simulink model "sensorMCU"  (Simulink 6.6)
settings: Solver=FixedStepDiscrete  StartTime=0.0  StopTime=10.0  FixedStep=0.01  RelTol=1e-3
InitFcn:
  | mcuInit
values from neighbouring files (symbols this model uses):
  gxGainrad = gxGain*pi/180    [mcuInit.m]
  gyGainrad = gyGain*pi/180    [mcuInit.m]
  gzGainrad = gzGain*pi/180    [mcuInit.m]
  T = 0.01    [initGPS.m]    (also in mcuInit.m)
undefined symbols (not defined in the file or in its folder): AccelParam, floatToBytes, gaind, gpsInit, gpsParse, gpsRead, gpsSeparate, gyTGain, hil_getEuler, hil_getGPSRead, hil_getRates, hil_getRawRead, hil_getVned, hil_getXYZ, hilRead, logData, loggerInit, MagParam, mzTGain, polesd, protParseDecode, protParserInit, shortToBytes, spiMasterInit, spiSend, stTGain, tmeanMz, tmeanSt, tmeanVl, u1, uartInit, uShortToBytes, vlTGain, y1, zerosd
libraries: dsPICdrivers x72, simulink x6, dspswit3 x1, dspsigops x1, xpclib x1, aerolibconvert2 x1
(part 1 of 3)
settings Model: Creator=ASL_Lab  LastModifiedBy=Administrator  BufferReuse=off  ProdHWDeviceType=16-bit Generic
settings OptimizationCC: BlockReduction=off  InlineParams=on  OptimizeBlockIOStorage=off  BufferReuse=off  ExpressionFolding=off  LocalBlockOutputs=off  EfficientFloat2IntCast=on  OptimizeModelRefInitCode=on  LifeSpan=1
settings HardwareCC: ProdBitPerInt=16  ProdEndianess=LittleEndian  ProdWordSize=16  ProdHWDeviceType=16-bit Generic  TargetHWDeviceType=32-bit Generic
settings RTWCC: SystemTargetFile=dspic.tlc  TemplateMakefile=dspic_pic30_gcc.tmf  PostCodeGenCommand=dsPIC_Compile()  Description=Embedded Target for Microchip dsPIC (real-time)  GenerateReport=on  ProcessScript=dspic_make_rtw_hook  CustomHeaderCode="#include \"apDefinitions.h\""  IncludeHyperlinkInReport=on  LaunchReport=on
settings RTWCC: CustomSource=|
  | clib\circBuffer.c
  | clib\gpsParse.c
  | clib\gpsSplit.c
  | clib\sbrk.c
  | clib\bufferedUART.c
  | clib\dataLogger.c
  | clib\interProcCommMaster.c
  | clib\conversions.c
  | clib\apUtils.c
  | clib\protDecoder.c
settings CodeAppCC: IgnoreCustomStorageClasses=off
settings STFCustomTargetCC: TargetFcnLib=ansi_tfl_tmw.mat  GenFloatMathFcnCalls=ANSI_C  ModelReferenceCompliant=off  IncludeMdlTerminateFcn=off  CombineOutputUpdateFcns=on  SuppressErrorStatus=on  ERTCustomFileBanners=on  SupportContinuousTime=off  SupportNonInlinedSFcns=off  SystemTargetFile=dspic.tlc
settings ERTTargetCC: TargetFcnLib=ansi_tfl_tmw.mat  GenFloatMathFcnCalls=ANSI_C  ModelReferenceCompliant=off  IncludeMdlTerminateFcn=off  SuppressErrorStatus=on  ModelStepFunctionPrototypeControlCompliant=off  ExtModeMexFile=noextcomm  InlinedParameterPlacement=NonHierarchical  ERTSrcFileBannerTemplate=dsPIC_code_template.cgt  ERTHdrFileBannerTemplate=dsPIC_code_template.cgt  ERTDataSrcFileTemplate=dsPIC_code_template.cgt  ERTDataHdrFileTemplate=dsPIC_code_template.cgt  ERTCustomFileTemplate=dsPIC_main.tlc
settings CustomProperty: DataType=string  Value=C:\PROGRA~1\MATLAB\R2007a\rtw\bin\win32\gmake

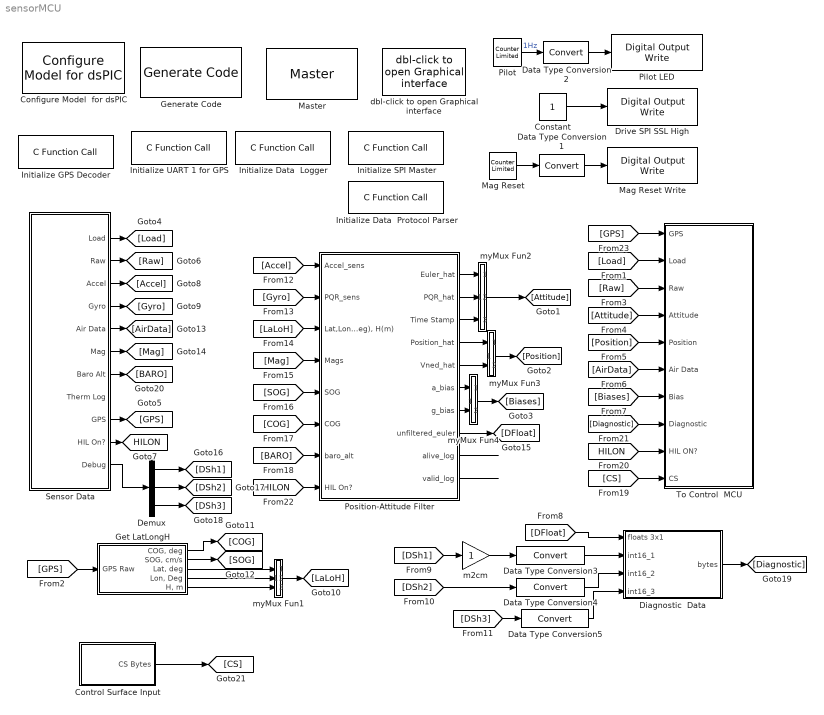
== system sensorMCU ==
  Configure Model  for dsPIC : dsPICdrivers/Simulink Configuration/Configure Model  for dsPIC
  Constant : Constant  OutDataTypeMode=boolean
  Control Surface Input : Subsystem
  Data Type Conversion1 : DataTypeConversion  OutDataTypeMode=boolean
  Data Type Conversion2 : DataTypeConversion  OutDataTypeMode=boolean
  Data Type Conversion3 : DataTypeConversion  OutDataTypeMode=int16
  Data Type Conversion4 : DataTypeConversion  OutDataTypeMode=int16
  Data Type Conversion5 : DataTypeConversion  OutDataTypeMode=int16
  Demux : Demux  Outputs=3
  Diagnostic  Data : Subsystem
  Drive SPI SSL High : dsPICdrivers/Digital I//O/Digital Output Write  Tag=dsPIC_Digital_Output  Priority=5  PORT=B  Pin=[ 2]  Simultaneous=off  OrderingInOutPopup=None
  Generate Code : dsPICdrivers/Simulink Configuration/Generate Code
  Get LatLongH : Subsystem
  Initialize Data  Logger : dsPICdrivers/OTHERS/C Function Call  Tag=dsPIC_dsPIC_CFunctionCall  fctName='loggerInit'  INPUT_SIZE=1  INPUT1=--  INPUT2=--  INPUT3=--  OUTPUT_SIZE=1  OUTPUT1=--  SampleTime=inf  InputType=[ ]  OutputType=[ ]  FctDeclaration=extern void loggerInit();  FctCall=loggerInit();  OrderingInOutPopup=None
  Initialize Data  Protocol Parser : dsPICdrivers/OTHERS/C Function Call  Tag=dsPIC_dsPIC_CFunctionCall  fctName='protParserInit'  INPUT_SIZE=1  INPUT1=--  INPUT2=--  INPUT3=--  OUTPUT_SIZE=1  OUTPUT1=--  SampleTime=inf  InputType=[ ]  OutputType=[ ]  FctDeclaration=extern void protParserInit();  FctCall=protParserInit();  OrderingInOutPopup=None
  Initialize GPS Decoder : dsPICdrivers/OTHERS/C Function Call  Tag=dsPIC_dsPIC_CFunctionCall  fctName='gpsInit'  INPUT_SIZE=1  INPUT1=--  INPUT2=--  INPUT3=--  OUTPUT_SIZE=1  OUTPUT1=--  SampleTime=inf  InputType=[ ]  OutputType=[ ]  FctDeclaration=extern void gpsInit();  FctCall=gpsInit();  OrderingInOutPopup=None
  Initialize SPI Master : dsPICdrivers/OTHERS/C Function Call  Tag=dsPIC_dsPIC_CFunctionCall  fctName='spiMasterInit'  INPUT_SIZE=1  INPUT1=--  INPUT2=--  INPUT3=--  OUTPUT_SIZE=1  OUTPUT1=--  SampleTime=inf  InputType=[ ]  OutputType=[ ]  FctDeclaration=extern void spiMasterInit();  FctCall=spiMasterInit();  OrderingInOutPopup=None
  Initialize UART 1 for GPS : dsPICdrivers/OTHERS/C Function Call  Tag=dsPIC_dsPIC_CFunctionCall  fctName='uartInit'  INPUT_SIZE=1  INPUT1=--  INPUT2=--  INPUT3=--  OUTPUT_SIZE=1  OUTPUT1=--  SampleTime=inf  InputType=[ ]  OutputType=[ ]  FctDeclaration=extern void uartInit();  FctCall=uartInit();  OrderingInOutPopup=None
  Mag Reset : simulink/Sources/Counter Limited  SystemSampleTime=-1  uplimit=1  tsamp=.01
  Mag Reset Write : dsPICdrivers/Digital I//O/Digital Output Write  Tag=dsPIC_Digital_Output  Priority=5  PORT=G  Pin=[12]  Simultaneous=off  OrderingInOutPopup=None
  Master : dsPICdrivers/Master  Tag=dsPIC_MASTER  Priority=1  TimeStepType=Timer1  picType=33fJ256MC710  fcy=40000000  Quartz_33f=12e6  PLLActive_33f=on  fcyDesired_33f=40e6  tmr1="[8  49999  0]"  tmr1Info="Time Step : 0.01  ;   Error : 0%  PR1=49999"  tmr2345="[8  0  0  0  0  0  0  0]"  tmr2345cfg=[-1 -1 -1 -1 -1 -1 -1 -1]  IOautoConf=on  typePort="[ 0   0   0   0   0   0   0   0   0   0   0   0   0   0   9   9   8   8  10   8   8   8   8   8   8   8   8   8   8   8   0   8   0   8   0   0   0   0   0   0   0   0   0   0   0   0   0   0   0   0   9   0   0   0   0   0   0   6   6   6   6   6   0   0   0   0   0   0   0   0   0   0   0   0   0   0   0   0   0   0   0   0   0   0   0   0   0   0   0   0   0   0   0   0   0   0   0   0   0   0   0   0   0   0   0   0   0   0  10   0  10   0 ]"  TRIS="[ 65535  65531  65535  65535  65535  65535  45055 ]"  ADPCFG=4  MasterBusyPort=None  MasterOverloadPort=None  FOSC=Quartz (XT - HS)  TempProtection_33f=TEMP_ON  FPBOR=<empty>  PWRT=64ms  MCLR=<empty>  PowerSave=off
  Pilot : simulink/Sources/Counter Limited  SystemSampleTime=-1  uplimit=1  tsamp=1.0
  Pilot LED : dsPICdrivers/Digital I//O/Digital Output Write  Tag=dsPIC_Digital_Output  Priority=5  PORT=G  Pin=[14]  Simultaneous=off  OrderingInOutPopup=None
  Position-Attitude Filter : Subsystem
  Sensor Data : Subsystem
  To Control  MCU : Subsystem
  dbl-click to open Graphical interface : dsPICdrivers/Serial PORT/dbl-click to open Graphical interface  SystemSampleTime=-1  Nothing=0
  m2cm : Gain
  myMux Fun1 : Stateflow chart
  myMux Fun2 : Stateflow chart
  myMux Fun3 : Stateflow chart
  myMux Fun4 : Stateflow chart
  tag scope: HILON=global
  wires:
  Pilot/1 -> Data Type Conversion2/1  "1Hz"
  Data Type Conversion2/1 -> Pilot LED/1
  Constant/1 -> Drive SPI SSL High/1
  myMux Fun1/1(y) -> [LaLoH]
  Mag Reset/1 -> Data Type Conversion1/1
  Data Type Conversion1/1 -> Mag Reset Write/1
  m2cm/1 -> Data Type Conversion3/1
  [Biases] -> To Control  MCU/7(Bias)
  [Diagnostic] -> To Control  MCU/8(Diagnostic)
  [GPS] -> To Control  MCU/1(GPS)
  Position-Attitude Filter/3(Time Stamp) -> myMux Fun2/3(u3)
  Position-Attitude Filter/5(Vned_hat) -> myMux Fun3/2(u2)
  Position-Attitude Filter/6(a_bias) -> myMux Fun4/1(u1)
  Position-Attitude Filter/7(g_bias) -> myMux Fun4/2(u2)
  myMux Fun2/1(y) -> [Attitude]
  myMux Fun3/1(y) -> [Position]
  myMux Fun4/1(y) -> [Biases]
  Sensor Data/1(Load) -> [Load]
  [Load] -> To Control  MCU/2(Load)
  [GPS] -> Get LatLongH/1(GPS Raw)
  [Raw] -> To Control  MCU/3(Raw)
  Get LatLongH/3("Lat, deg") -> myMux Fun1/1(u1)
  Get LatLongH/4("Lon, Deg") -> myMux Fun1/2(u2)
  Get LatLongH/5("H, m") -> myMux Fun1/3(u3)
  Get LatLongH/1("COG, deg") -> [COG]
  Get LatLongH/2("SOG, cm/s") -> [SOG]
  Sensor Data/2(Raw) -> [Raw]
  Sensor Data/3(Accel) -> [Accel]
  Sensor Data/4(Gyro) -> [Gyro]
  Sensor Data/5(Air Data) -> [AirData]
  Sensor Data/6(Mag) -> [Mag]
  Position-Attitude Filter/8(unfiltered_euler) -> [DFloat]
  [Attitude] -> To Control  MCU/4(Attitude)
  [Position] -> To Control  MCU/5(Position)
  [AirData] -> To Control  MCU/6(Air Data)
  Sensor Data/9(GPS) -> [GPS]
  Data Type Conversion3/1 -> Diagnostic  Data/2(int16_1)
  Data Type Conversion4/1 -> Diagnostic  Data/3(int16_2)
  Sensor Data/10(HIL On?) -> [HILON]
  Position-Attitude Filter/10(valid_log) -> ?
  [DFloat] -> Diagnostic  Data/1(floats 3x1)
  [DSh1] -> m2cm/1
  [DSh2] -> Data Type Conversion4/1
  [DSh3] -> Data Type Conversion5/1
  [HILON] -> To Control  MCU/9(HIL ON?)
  Diagnostic  Data/1(bytes) -> [Diagnostic]
  [Accel] -> Position-Attitude Filter/1(Accel_sens)
  [Gyro] -> Position-Attitude Filter/2(PQR_sens)
  [LaLoH] -> Position-Attitude Filter/3("Lat,Lon(deg), H(m)")
  [Mag] -> Position-Attitude Filter/4(Mags)
  [SOG] -> Position-Attitude Filter/5(SOG)
  [COG] -> Position-Attitude Filter/6(COG)
  Position-Attitude Filter/9(alive_log) -> ?
  Data Type Conversion5/1 -> Diagnostic  Data/4(int16_3)
  Sensor Data/11(Debug) -> Demux/1
  Demux/1 -> [DSh1]
  Demux/2 -> [DSh2]
  Demux/3 -> [DSh3]
  [BARO] -> Position-Attitude Filter/7(baro_alt)
  Sensor Data/7(Baro Alt) -> [BARO]
  Position-Attitude Filter/1(Euler_hat) -> myMux Fun2/1(u1)
  Position-Attitude Filter/2(PQR_hat) -> myMux Fun2/2(u2)
  Position-Attitude Filter/4(Position_hat) -> myMux Fun3/1(u1)
  Control Surface Input/1(CS Bytes) -> [CS]
  [CS] -> To Control  MCU/10(CS)
  [HILON] -> Position-Attitude Filter/8(HIL On?)

== system sensorMCU/Control Surface Input ==
  C Function Call{1..5} (5 alike) : dsPICdrivers/OTHERS/C Function Call  Tag=dsPIC_dsPIC_CFunctionCall  fctName='uShortToBytes'  INPUT_SIZE=1  INPUT1=uint16  INPUT2=--  INPUT3=--  OUTPUT_SIZE=2  OUTPUT1=uint8  SampleTime=-1  InputType=[ 4 ]  OutputType=[ 2 ]  FctDeclaration=extern void uShortToBytes(uint16_T u1,uint8_T* y1);  FctCall=uShortToBytes(%u1, *%y1);  OrderingInOutPopup=None
  Input Capture : dsPICdrivers/Peripheral I//O/Input Capture  Tag=dsPIC_PWM_IC  Priority=5  IntPriority=6  Channel=[ 2 3 4 5 6]  Channel_UP_Down_Periode="[1  1  1  1  1]"  MaxChannel="[0.0025      0.0025      0.0025      0.0025      0.0025]"  SafeMarge="[10  10  10  10  10]"  MaxName=' IC2max , IC3max , IC4max , IC5max , IC6max '  Precision="[13.6096      13.6096      13.6096      13.6096      13.6096]"  Timer="[2  2  2  2  2]"  ChangeDetected="[0  0  0  0  0]"  ChangeDetectedPortRef=3  SampleTime=.01  Status=OK
  myMux Fun5 : Stateflow chart
  CS Bytes : Outport
  wires:
  Input Capture/1 -> C Function Call2/1
  Input Capture/2 -> C Function Call1/1
  Input Capture/3 -> C Function Call3/1
  Input Capture/4 -> C Function Call4/1
  Input Capture/5 -> C Function Call5/1
  C Function Call2/1 -> myMux Fun5/1(u1)
  C Function Call1/1 -> myMux Fun5/2(u2)
  C Function Call3/1 -> myMux Fun5/3(u3)
  C Function Call4/1 -> myMux Fun5/4(u4)
  C Function Call5/1 -> myMux Fun5/5(u5)
  myMux Fun5/1(y) -> CS Bytes/1

== system sensorMCU/Diagnostic  Data ==
  floats 3x1 : Inport
  int16_1 : Inport  Port=2
  int16_2 : Inport  Port=3
  int16_3 : Inport  Port=4
  C Function Call : dsPICdrivers/OTHERS/C Function Call  Tag=dsPIC_dsPIC_CFunctionCall  fctName='shortToBytes'  INPUT_SIZE=1  INPUT1=int16  INPUT2=--  INPUT3=--  OUTPUT_SIZE=2  OUTPUT1=uint8  SampleTime=-1  InputType=[ 3 ]  OutputType=[ 2 ]  FctDeclaration=extern void shortToBytes(int16_T u1,uint8_T* y1);  FctCall=shortToBytes(%u1, *%y1);  OrderingInOutPopup=None
  C Function Call1 : dsPICdrivers/OTHERS/C Function Call  Tag=dsPIC_dsPIC_CFunctionCall  fctName='shortToBytes'  INPUT_SIZE=1  INPUT1=int16  INPUT2=--  INPUT3=--  OUTPUT_SIZE=2  OUTPUT1=uint8  SampleTime=-1  InputType=[ 3 ]  OutputType=[ 2 ]  FctDeclaration=extern void shortToBytes(int16_T u1,uint8_T* y1);  FctCall=shortToBytes(%u1, *%y1);  OrderingInOutPopup=None
  C Function Call2 : dsPICdrivers/OTHERS/C Function Call  Tag=dsPIC_dsPIC_CFunctionCall  fctName='shortToBytes'  INPUT_SIZE=1  INPUT1=int16  INPUT2=--  INPUT3=--  OUTPUT_SIZE=2  OUTPUT1=uint8  SampleTime=-1  InputType=[ 3 ]  OutputType=[ 2 ]  FctDeclaration=extern void shortToBytes(int16_T u1,uint8_T* y1);  FctCall=shortToBytes(%u1, *%y1);  OrderingInOutPopup=None
  myMux Fun2 : Stateflow chart
  to Bytes6 : Subsystem
  bytes : Outport
  wires:
  to Bytes6/1(Bytes) -> myMux Fun2/1(u1)
  C Function Call/1 -> myMux Fun2/2(u2)
  C Function Call1/1 -> myMux Fun2/3(u3)
  floats 3x1/1 -> to Bytes6/1(Float)
  int16_1/1 -> C Function Call/1
  myMux Fun2/1(y) -> bytes/1
  int16_2/1 -> C Function Call1/1
  int16_3/1 -> C Function Call2/1
  C Function Call2/1 -> myMux Fun2/4(u4)

== system sensorMCU/Get LatLongH ==
  GPS Raw : Inport
  C Function Call : dsPICdrivers/OTHERS/C Function Call  Tag=dsPIC_dsPIC_CFunctionCall  fctName='bytesToFloat'  INPUT_SIZE=4  INPUT1=uint8  INPUT2=--  INPUT3=--  OUTPUT_SIZE=1  OUTPUT1=real32  SampleTime=-1  InputType=[ 2 ]  OutputType=[ 7 ]  FctDeclaration=extern real32_T bytesToFloat(uint8_T* u1);  FctCall=%y1 = bytesToFloat(*%u1);  OrderingInOutPopup=None
  C Function Call1 : dsPICdrivers/OTHERS/C Function Call  Tag=dsPIC_dsPIC_CFunctionCall  fctName='bytesToFloat'  INPUT_SIZE=4  INPUT1=uint8  INPUT2=--  INPUT3=--  OUTPUT_SIZE=1  OUTPUT1=real32  SampleTime=-1  InputType=[ 2 ]  OutputType=[ 7 ]  FctDeclaration=extern real32_T bytesToFloat(uint8_T* u1);  FctCall=%y1 = bytesToFloat(*%u1);  OrderingInOutPopup=None
  C Function Call2 : dsPICdrivers/OTHERS/C Function Call  Tag=dsPIC_dsPIC_CFunctionCall  fctName='bytesToFloat'  INPUT_SIZE=4  INPUT1=uint8  INPUT2=--  INPUT3=--  OUTPUT_SIZE=1  OUTPUT1=real32  SampleTime=-1  InputType=[ 2 ]  OutputType=[ 7 ]  FctDeclaration=extern real32_T bytesToFloat(uint8_T* u1);  FctCall=%y1 = bytesToFloat(*%u1);  OrderingInOutPopup=None
  C Function Call3 : dsPICdrivers/OTHERS/C Function Call  Tag=dsPIC_dsPIC_CFunctionCall  fctName='bytesToUShort'  INPUT_SIZE=2  INPUT1=uint8  INPUT2=--  INPUT3=--  OUTPUT_SIZE=1  OUTPUT1=uint16  SampleTime=-1  InputType=[ 2 ]  OutputType=[ 4 ]  FctDeclaration=extern uint16_T bytesToUShort(uint8_T* u1);  FctCall=%y1 = bytesToUShort(*%u1);  OrderingInOutPopup=None
  C Function Call4 : dsPICdrivers/OTHERS/C Function Call  Tag=dsPIC_dsPIC_CFunctionCall  fctName='bytesToUShort'  INPUT_SIZE=2  INPUT1=uint8  INPUT2=--  INPUT3=--  OUTPUT_SIZE=1  OUTPUT1=uint16  SampleTime=-1  InputType=[ 2 ]  OutputType=[ 4 ]  FctDeclaration=extern uint16_T bytesToUShort(uint8_T* u1);  FctCall=%y1 = bytesToUShort(*%u1);  OrderingInOutPopup=None
  Demux : Demux  Outputs=[6 4 4 4 2 2 5]
  Terminator : Terminator
  Terminator1 : Terminator
  "COG, deg" : Outport
  "SOG, cm/s" : Outport  Port=2
  "Lat, deg" : Outport  Port=3
  "Lon, Deg" : Outport  Port=4
  "H, m" : Outport  Port=5
  wires:
  GPS Raw/1 -> Demux/1
  C Function Call/1 -> "Lat, deg"/1
  C Function Call1/1 -> "Lon, Deg"/1
  C Function Call2/1 -> "H, m"/1
  Demux/1 -> Terminator/1
  Demux/2 -> C Function Call/1
  Demux/3 -> C Function Call1/1
  Demux/4 -> C Function Call2/1
  Demux/7 -> Terminator1/1
  Demux/5 -> C Function Call3/1
  Demux/6 -> C Function Call4/1
  C Function Call3/1 -> "COG, deg"/1
  C Function Call4/1 -> "SOG, cm/s"/1

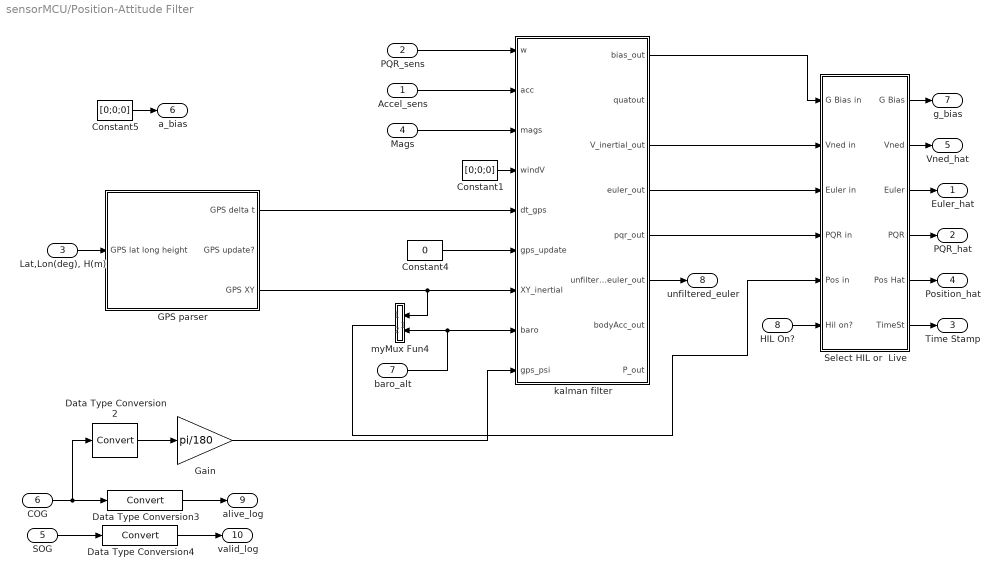
== system sensorMCU/Position-Attitude Filter ==
  Accel_sens : Inport
  PQR_sens : Inport  Port=2
  "Lat,Lon(deg), H(m)" : Inport  Port=3
  Mags : Inport  Port=4
  SOG : Inport  Port=5
  COG : Inport  Port=6
  baro_alt : Inport  Port=7
  HIL On? : Inport  Port=8
  Constant1 : Constant  Value=[0;0;0]
  Constant4 : Constant  Value=0
  Constant5 : Constant  Value=[0;0;0]
  Data Type Conversion2 : DataTypeConversion  OutDataTypeMode=double
  Data Type Conversion3 : DataTypeConversion  OutDataTypeMode=int16
  Data Type Conversion4 : DataTypeConversion  OutDataTypeMode=int16
  GPS parser : Subsystem
  Gain : Gain  Gain=pi/180
  Select HIL or  Live : Subsystem
  kalman filter : Stateflow chart
  myMux Fun4 : Stateflow chart  Orientation=left
  Euler_hat : Outport
  PQR_hat : Outport  Port=2
  Time Stamp : Outport  Port=3
  Position_hat : Outport  Port=4
  Vned_hat : Outport  Port=5
  a_bias : Outport  Port=6
  g_bias : Outport  Port=7
  unfiltered_euler : Outport  Port=8
  alive_log : Outport  Port=9
  valid_log : Outport  Port=10
  wires:
  "Lat,Lon(deg), H(m)"/1 -> GPS parser/1(GPS lat long height)
  Data Type Conversion3/1 -> alive_log/1
  Data Type Conversion4/1 -> valid_log/1
  COG/1 -> Data Type Conversion3/1, Data Type Conversion2/1
  SOG/1 -> Data Type Conversion4/1
  Data Type Conversion2/1 -> Gain/1
  Select HIL or  Live/4(PQR) -> PQR_hat/1
  Select HIL or  Live/3(Euler) -> Euler_hat/1
  PQR_sens/1 -> kalman filter/1(w)
  Accel_sens/1 -> kalman filter/2(acc)
  Mags/1 -> kalman filter/3(mags)
  Select HIL or  Live/1(G Bias) -> g_bias/1
  kalman filter/1(bias_out) -> Select HIL or  Live/1(G Bias in)
  kalman filter/4(euler_out) -> Select HIL or  Live/3(Euler in)
  kalman filter/5(pqr_out) -> Select HIL or  Live/4(PQR in)
  Constant1/1 -> kalman filter/4(windV)
  Constant5/1 -> a_bias/1
  kalman filter/3(V_inertial_out) -> Select HIL or  Live/2(Vned in)
  Select HIL or  Live/2(Vned) -> Vned_hat/1
  GPS parser/1(GPS delta t) -> kalman filter/5(dt_gps)
  myMux Fun4/1(y) -> Select HIL or  Live/5(Pos in)
  Select HIL or  Live/5(Pos Hat) -> Position_hat/1
  Gain/1 -> kalman filter/9(gps_psi)
  GPS parser/3(GPS XY) -> kalman filter/7(XY_inertial), myMux Fun4/1(u1)
  baro_alt/1 -> kalman filter/8(baro), myMux Fun4/2(u2)
  kalman filter/6(unfiltered_euler_out) -> unfiltered_euler/1
  Constant4/1 -> kalman filter/6(gps_update)
  HIL On?/1 -> Select HIL or  Live/6(Hil on?)
  Select HIL or  Live/6(TimeSt) -> Time Stamp/1

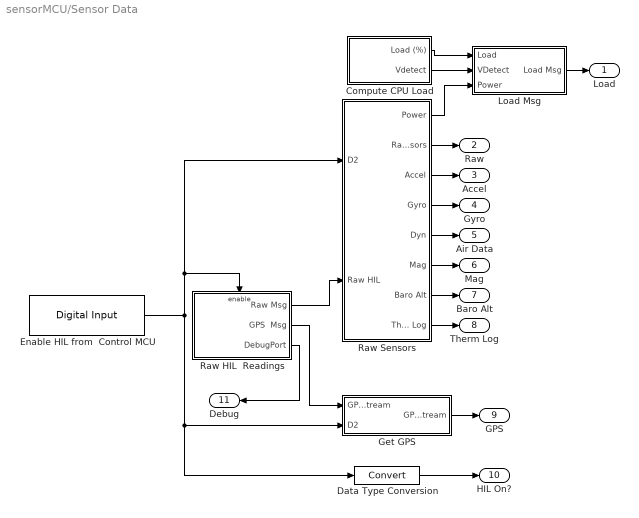
== system sensorMCU/Sensor Data ==
  Compute CPU Load : Subsystem
  Data Type Conversion : DataTypeConversion  OutDataTypeMode=uint8  SampleTime=0.01
  Enable HIL from  Control MCU : dsPICdrivers/Digital I//O/Digital Input  Tag=dsPIC_Digital_Input  PORT=D  Pin=[2]  SampleTime=.01  OrderingInOutPopup=None
  Get GPS : Subsystem
  Load Msg : Subsystem
  Raw HIL  Readings : Subsystem
  Raw Sensors : Subsystem
  Load : Outport
  Raw : Outport  Port=2
  Accel : Outport  Port=3
  Gyro : Outport  Port=4
  Air Data : Outport  Port=5
  Mag : Outport  Port=6
  Baro Alt : Outport  Port=7
  Therm Log : Outport  Port=8
  GPS : Outport  Port=9
  HIL On? : Outport  Port=10
  Debug : Outport  Orientation=left  Port=11
  wires:
  Compute CPU Load/1(Load (%)) -> Load Msg/1(Load)
  Compute CPU Load/2(Vdetect) -> Load Msg/2(VDetect)
  Raw Sensors/1(Power) -> Load Msg/3(Power)
  Load Msg/1(Load Msg) -> Load/1
  Raw Sensors/2(Raw Sensors) -> Raw/1
  Raw Sensors/3(Accel) -> Accel/1
  Raw Sensors/4(Gyro) -> Gyro/1
  Raw Sensors/5(Dyn) -> Air Data/1
  Raw Sensors/6(Mag) -> Mag/1
  Raw Sensors/7(Baro Alt) -> Baro Alt/1
  Raw Sensors/8(Therm Log) -> Therm Log/1
  Get GPS/1(GPS Stream) -> GPS/1
  Raw HIL  Readings/1(Raw Msg) -> Raw Sensors/2(Raw HIL)
  Raw HIL  Readings/2(GPS  Msg) -> Get GPS/1(GPS HIL Stream)
  Enable HIL from  Control MCU/1 -> Raw HIL  Readings/Enable, Raw Sensors/1(D2), Get GPS/2(D2), Data Type Conversion/1
  Data Type Conversion/1 -> HIL On?/1
  Raw HIL  Readings/3(DebugPort) -> Debug/1

== system sensorMCU/To Control  MCU ==
  GPS : Inport
  Load : Inport  Port=2
  Raw : Inport  Port=3
  Attitude : Inport  Port=4
  Position : Inport  Port=5
  Air Data : Inport  Port=6
  Bias : Inport  Port=7
  Diagnostic : Inport  Port=8
  HIL ON? : Inport  Port=9
  CS : Inport  Port=10
  Data Logger : dsPICdrivers/OTHERS/C Function Call  Tag=dsPIC_dsPIC_CFunctionCall  fctName='logData'  INPUT_SIZE=162  INPUT1=uint8  INPUT2=--  INPUT3=--  OUTPUT_SIZE=99  OUTPUT1=uint8  SampleTime=-1  InputType=[ 2 ]  OutputType=[ 2 ]  FctDeclaration=extern void logData(uint8_T* u1,uint8_T* y1);  FctCall=logData(*%u1, *%y1);  OrderingInOutPopup=None
  IPC Data : Subsystem
  myMux Fun : Stateflow chart
  wires:
  myMux Fun/1(y) -> Data Logger/1
  Data Logger/1 -> IPC Data/1(To SPI)
  GPS/1 -> myMux Fun/1(u1)
  Load/1 -> myMux Fun/2(u2)
  Raw/1 -> myMux Fun/3(u3)
  Attitude/1 -> myMux Fun/4(u4)
  Position/1 -> myMux Fun/5(u5)
  Air Data/1 -> myMux Fun/6(u6)
  Bias/1 -> myMux Fun/7(u7)
  Diagnostic/1 -> myMux Fun/8(u8)
  HIL ON?/1 -> myMux Fun/9(u9)
  CS/1 -> myMux Fun/10(u10)

== system sensorMCU/Diagnostic  Data/to Bytes6 ==
  Float : Inport
  C Function Call : dsPICdrivers/OTHERS/C Function Call  Tag=dsPIC_dsPIC_CFunctionCall  fctName='floatToBytes'  INPUT_SIZE=1  INPUT1=real32  INPUT2=--  INPUT3=--  OUTPUT_SIZE=4  OUTPUT1=uint8  SampleTime=-1  InputType=[ 7 ]  OutputType=[ 2 ]  FctDeclaration=extern void floatToBytes(real32_T u1,uint8_T* y1);  FctCall=floatToBytes(%u1, *%y1);  OrderingInOutPopup=None
  C Function Call1 : dsPICdrivers/OTHERS/C Function Call  Tag=dsPIC_dsPIC_CFunctionCall  fctName='floatToBytes'  INPUT_SIZE=1  INPUT1=real32  INPUT2=--  INPUT3=--  OUTPUT_SIZE=4  OUTPUT1=uint8  SampleTime=-1  InputType=[ 7 ]  OutputType=[ 2 ]  FctDeclaration=extern void floatToBytes(real32_T u1,uint8_T* y1);  FctCall=floatToBytes(%u1, *%y1);  OrderingInOutPopup=None
  C Function Call2 : dsPICdrivers/OTHERS/C Function Call  Tag=dsPIC_dsPIC_CFunctionCall  fctName='floatToBytes'  INPUT_SIZE=1  INPUT1=real32  INPUT2=--  INPUT3=--  OUTPUT_SIZE=4  OUTPUT1=uint8  SampleTime=-1  InputType=[ 7 ]  OutputType=[ 2 ]  FctDeclaration=extern void floatToBytes(real32_T u1,uint8_T* y1);  FctCall=floatToBytes(%u1, *%y1);  OrderingInOutPopup=None
  Data Type Conversion : DataTypeConversion  OutDataTypeMode=single
  Demux : Demux  Outputs=3
  Mux : Mux  Inputs=3
  Bytes : Outport
  wires:
  Float/1 -> Data Type Conversion/1
  Demux/1 -> C Function Call/1
  Mux/1 -> Bytes/1
  C Function Call/1 -> Mux/1
  Demux/2 -> C Function Call1/1
  Demux/3 -> C Function Call2/1
  C Function Call1/1 -> Mux/2
  C Function Call2/1 -> Mux/3
  Data Type Conversion/1 -> Demux/1

== system sensorMCU/Position-Attitude Filter/GPS parser ==
  GPS lat long height : Inport
  Constant : Constant  Orientation=left  Value=[0 , 37.0004768371582, -122.061897277832]
  Data Type Conversion : DataTypeConversion  OutDataTypeMode=double
  Demux : Demux  Outputs=3
  Demux1 : Demux  Outputs=3
  GPS Update : Subsystem
  Geod2LTP2 : Subsystem
      mask Description:
      | This block provides transformation of the Geodetic coordinates
      | to the LTP coorinate system. The block uses two consecutive transformations
      | (Geodetic -> ECEF ->LTP).
      | Geodetic coordinates of the LTP origin should also be predetermined.
      mask Help: Oops!
      mask Display: plot(0,0,100,100,[45,40,35,40,40],[85,95,85,95,40],[85,95,85,95,40],[35,40,45,40,40],[60,40,10,20,10,14],[70,40,10,13,10,20],[56,45],[70,70],[60,60],[50,60],[60,60],[30,40],[50,60],[20,20],[30,40],[20,20],[45,55],[35,25],[75,65],[35,25])
  Mux2 : Mux  Inputs=2
  GPS delta t : Outport
  GPS update? : Outport  Port=2
  GPS XY : Outport  Port=3
  wires:
  Mux2/1 -> GPS XY/1
  Demux1/2 -> Mux2/2
  Demux1/1 -> Mux2/1
  GPS Update/1(Update?) -> GPS update?/1
  GPS Update/2(delta t) -> GPS delta t/1
  Constant/1 -> Geod2LTP2/1("Height, Lat, Lon Initials from GPS")
  Geod2LTP2/1("NEU, m") -> Demux1/1, GPS Update/1(XYZ)
  Demux/1 -> Geod2LTP2/2("Lat, deg(GPS)")
  Demux/2 -> Geod2LTP2/3("Lon, deg(GPS)")
  Demux/3 -> Geod2LTP2/4(Hight,m(GPS))
  GPS lat long height/1 -> Data Type Conversion/1
  Data Type Conversion/1 -> Demux/1

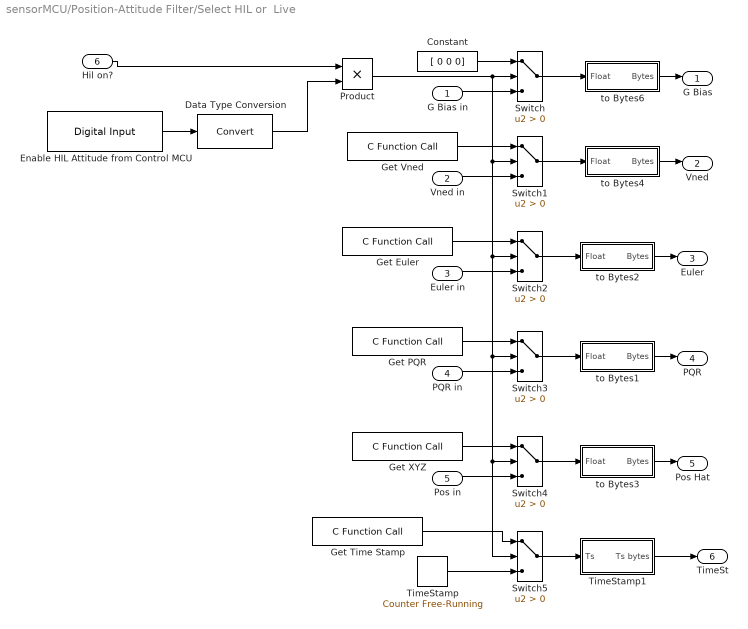
== system sensorMCU/Position-Attitude Filter/Select HIL or  Live ==
  G Bias in : Inport
  Vned in : Inport  Port=2
  Euler in : Inport  Port=3
  PQR in : Inport  Port=4
  Pos in : Inport  Port=5
  Hil on? : Inport  Port=6
  Constant : Constant  Value=[ 0 0 0]  OutDataTypeMode=single
  Data Type Conversion : DataTypeConversion  OutDataTypeMode=uint8
  Enable HIL Attitude from Control MCU : dsPICdrivers/Digital I//O/Digital Input  Tag=dsPIC_Digital_Input  PORT=A  Pin=[14]  SampleTime=.01  OrderingInOutPopup=None
  Get Euler : dsPICdrivers/OTHERS/C Function Call  Tag=dsPIC_dsPIC_CFunctionCall  fctName='hil_getEuler'  INPUT_SIZE=1  INPUT1=--  INPUT2=--  INPUT3=--  OUTPUT_SIZE=3  OUTPUT1=real32  SampleTime=.01  InputType=[ ]  OutputType=[ 7 ]  FctDeclaration=extern void hil_getEuler(real32_T* y1);  FctCall=hil_getEuler(*%y1);  OrderingInOutPopup=None
  Get PQR : dsPICdrivers/OTHERS/C Function Call  Tag=dsPIC_dsPIC_CFunctionCall  fctName='hil_getRates'  INPUT_SIZE=1  INPUT1=--  INPUT2=--  INPUT3=--  OUTPUT_SIZE=3  OUTPUT1=real32  SampleTime=.01  InputType=[ ]  OutputType=[ 7 ]  FctDeclaration=extern void hil_getRates(real32_T* y1);  FctCall=hil_getRates(*%y1);  OrderingInOutPopup=None
  Get Time Stamp : dsPICdrivers/OTHERS/C Function Call  Tag=dsPIC_dsPIC_CFunctionCall  fctName='hil_getTs'  INPUT_SIZE=1  INPUT1=--  INPUT2=--  INPUT3=--  OUTPUT_SIZE=1  OUTPUT1=uint16  SampleTime=.01  InputType=[ ]  OutputType=[ 4 ]  FctDeclaration=extern uint16_T hil_getTs();  FctCall=%y1 = hil_getTs();  OrderingInOutPopup=None
  Get Vned : dsPICdrivers/OTHERS/C Function Call  Tag=dsPIC_dsPIC_CFunctionCall  fctName='hil_getVned'  INPUT_SIZE=1  INPUT1=--  INPUT2=--  INPUT3=--  OUTPUT_SIZE=3  OUTPUT1=real32  SampleTime=.01  InputType=[ ]  OutputType=[ 7 ]  FctDeclaration=extern void hil_getVned(real32_T* y1);  FctCall=hil_getVned(*%y1);  OrderingInOutPopup=None
  Get XYZ : dsPICdrivers/OTHERS/C Function Call  Tag=dsPIC_dsPIC_CFunctionCall  fctName='hil_getXYZ'  INPUT_SIZE=1  INPUT1=--  INPUT2=--  INPUT3=--  OUTPUT_SIZE=3  OUTPUT1=real32  SampleTime=.01  InputType=[ ]  OutputType=[ 7 ]  FctDeclaration=extern void hil_getXYZ(real32_T* y1);  FctCall=hil_getXYZ(*%y1);  OrderingInOutPopup=None
  Product : Product  RndMeth=Zero
  Switch{,1..5} (6 alike) : Switch  Criteria=u2 > Threshold
  TimeStamp : simulink/Sources/Counter Free-Running  SystemSampleTime=-1  NumBits=16  tsamp=.01
  TimeStamp1 : Subsystem
  to Bytes1 : Subsystem
  to Bytes2 : Subsystem
  to Bytes3 : Subsystem
  to Bytes4 : Subsystem
  to Bytes6 : Subsystem
  G Bias : Outport
  Vned : Outport  Port=2
  Euler : Outport  Port=3
  PQR : Outport  Port=4
  Pos Hat : Outport  Port=5
  TimeSt : Outport  Port=6
  wires:
  to Bytes6/1(Bytes) -> G Bias/1
  to Bytes4/1(Bytes) -> Vned/1
  to Bytes2/1(Bytes) -> Euler/1
  to Bytes1/1(Bytes) -> PQR/1
  to Bytes3/1(Bytes) -> Pos Hat/1
  Switch/1 -> to Bytes6/1(Float)
  Constant/1 -> Switch/1
  Product/1 -> Switch/2, Switch1/2, Switch2/2, Switch3/2, Switch4/2, Switch5/2
  G Bias in/1 -> Switch/3
  Switch1/1 -> to Bytes4/1(Float)
  Get Vned/1 -> Switch1/1
  Vned in/1 -> Switch1/3
  Get Euler/1 -> Switch2/1
  Euler in/1 -> Switch2/3
  Switch2/1 -> to Bytes2/1(Float)
  Get PQR/1 -> Switch3/1
  PQR in/1 -> Switch3/3
  Switch3/1 -> to Bytes1/1(Float)
  Get XYZ/1 -> Switch4/1
  Pos in/1 -> Switch4/3
  Switch4/1 -> to Bytes3/1(Float)
  TimeStamp/1 -> Switch5/3
  Get Time Stamp/1 -> Switch5/1
  Enable HIL Attitude from Control MCU/1 -> Data Type Conversion/1
  Hil on?/1 -> Product/1
  Data Type Conversion/1 -> Product/2
  TimeStamp1/1(Ts bytes) -> TimeSt/1
  Switch5/1 -> TimeStamp1/1(Ts)

== system sensorMCU/Sensor Data/Compute CPU Load ==
  Calculus Time Step : dsPICdrivers/OTHERS/Calculus Time Step  Tag=dsPIC_CalculusTimeStep  SampleTime=0.01  PR1chk=on
  Data Type Conversion1 : DataTypeConversion  OutDataTypeMode=single
  Data Type Conversion12 : DataTypeConversion  OutDataTypeMode=uint8
  Data Type Conversion2 : DataTypeConversion  OutDataTypeMode=single
  Digital Input : dsPICdrivers/Digital I//O/Digital Input  Tag=dsPIC_Digital_Input  PORT=A  Pin=[15]  SampleTime=-1  OrderingInOutPopup=None
  Divide : Product  Inputs=*/  OutDataTypeMode=double  OutScaling=2^-10
  Gain : Gain  Gain=100
  Rounding Function : Rounding
  Load (%) : Outport
  Vdetect : Outport  Port=2
  wires:
  Calculus Time Step/1 -> Data Type Conversion2/1
  Calculus Time Step/2 -> Data Type Conversion1/1
  Divide/1 -> Gain/1
  Rounding Function/1 -> Data Type Conversion12/1
  Data Type Conversion1/1 -> Divide/2
  Data Type Conversion2/1 -> Divide/1
  Data Type Conversion12/1 -> Load (%)/1
  Digital Input/1 -> Vdetect/1
  Gain/1 -> Rounding Function/1

== system sensorMCU/Sensor Data/Get GPS ==
  GPS HIL Stream : Inport
  D2 : Inport  Port=2
  Logical Operator : Logic  Operator=NOT  AllPortsSameDT=off  OutDataTypeMode=Boolean
  Read GPS : Subsystem
  Switch : Switch
  GPS Stream : Outport
  wires:
  Switch/1 -> GPS Stream/1
  Read GPS/1(Out1) -> Switch/3
  Logical Operator/1 -> Read GPS/Enable
  D2/1 -> Switch/2, Logical Operator/1
  GPS HIL Stream/1 -> Switch/1

== system sensorMCU/Sensor Data/Load Msg ==
  Load : Inport
  VDetect : Inport  Port=2
  Power : Inport  Port=3
  C Function Call : dsPICdrivers/OTHERS/C Function Call  Tag=dsPIC_dsPIC_CFunctionCall  fctName='uShortToBytes'  INPUT_SIZE=1  INPUT1=uint16  INPUT2=--  INPUT3=--  OUTPUT_SIZE=4  OUTPUT1=uint8  SampleTime=-1  InputType=[ 4 ]  OutputType=[ 2 ]  FctDeclaration=extern void uShortToBytes(uint16_T u1,uint8_T* y1);  FctCall=uShortToBytes(%u1, *%y1);  OrderingInOutPopup=None
  myMux Fun : Stateflow chart
  Load Msg : Outport
  wires:
  Power/1 -> C Function Call/1
  C Function Call/1 -> myMux Fun/3(u3)
  VDetect/1 -> myMux Fun/2(u2)
  Load/1 -> myMux Fun/1(u1)
  myMux Fun/1(y) -> Load Msg/1

== system sensorMCU/Sensor Data/Raw HIL  Readings ==
  Enable : EnablePort
  Demux : Demux  Outputs=[3 3 97]
  Parser/Decoder : dsPICdrivers/OTHERS/C Function Call  Tag=dsPIC_dsPIC_CFunctionCall  fctName='protParseDecode'  INPUT_SIZE=103  INPUT1=uint8  INPUT2=--  INPUT3=--  OUTPUT_SIZE=1  OUTPUT1=--  SampleTime=-1  InputType=[ 2 ]  OutputType=[ ]  FctDeclaration=extern void protParseDecode(uint8_T* u1);  FctCall=protParseDecode(*%u1);  OrderingInOutPopup=Output
  Read Data from HIL : dsPICdrivers/OTHERS/C Function Call  Tag=dsPIC_dsPIC_CFunctionCall  fctName='hil_getRawRead'  INPUT_SIZE=1  INPUT1=--  INPUT2=--  INPUT3=--  OUTPUT_SIZE=15  OUTPUT1=uint16  SampleTime=0.01  InputType=[ ]  OutputType=[ 4 ]  FctDeclaration=extern void hil_getRawRead(uint16_T* y1);  FctCall=hil_getRawRead(*%y1);  OrderingInOutPopup=Input & Output
  Read Data from HIL1 : dsPICdrivers/OTHERS/C Function Call  Tag=dsPIC_dsPIC_CFunctionCall  fctName='hil_getGPSRead'  INPUT_SIZE=1  INPUT1=--  INPUT2=--  INPUT3=--  OUTPUT_SIZE=27  OUTPUT1=uint8  SampleTime=0.01  InputType=[ ]  OutputType=[ 2 ]  FctDeclaration=extern void hil_getGPSRead(uint8_T* y1);  FctCall=hil_getGPSRead(*%y1);  OrderingInOutPopup=Input
  Read Data from HIL2 : dsPICdrivers/OTHERS/C Function Call  Tag=dsPIC_dsPIC_CFunctionCall  fctName='hilRead'  INPUT_SIZE=1  INPUT1=--  INPUT2=--  INPUT3=--  OUTPUT_SIZE=103  OUTPUT1=uint8  SampleTime=0.01  InputType=[ ]  OutputType=[ 2 ]  FctDeclaration=extern void hilRead(uint8_T* y1);  FctCall=hilRead(*%y1);  OrderingInOutPopup=None
  Raw Msg : Outport
  GPS  Msg : Outport  Port=2
  DebugPort : Outport  Port=3
  wires:
  Read Data from HIL/1 -> Raw Msg/1
  Read Data from HIL/2 -> Read Data from HIL1/1
  Read Data from HIL1/1 -> GPS  Msg/1
  Demux/1 -> DebugPort/1
  Read Data from HIL2/1 -> Demux/1, Parser/Decoder/1
  Parser/Decoder/1 -> Read Data from HIL/1

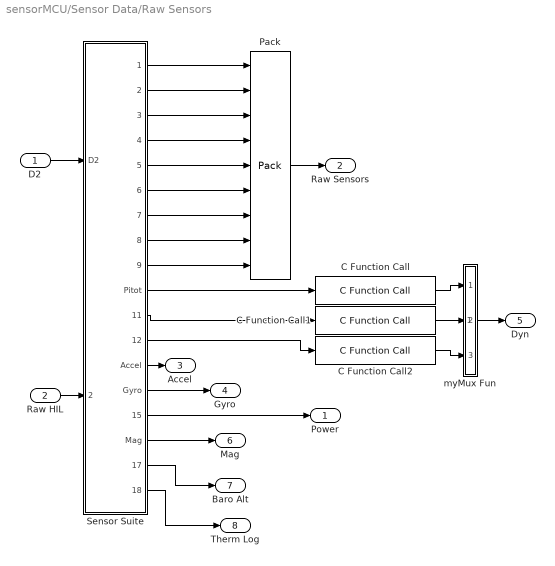
== system sensorMCU/Sensor Data/Raw Sensors ==
  D2 : Inport
  Raw HIL : Inport  Port=2
  C Function Call : dsPICdrivers/OTHERS/C Function Call  Tag=dsPIC_dsPIC_CFunctionCall  fctName='floatToBytes'  INPUT_SIZE=1  INPUT1=real32  INPUT2=--  INPUT3=--  OUTPUT_SIZE=4  OUTPUT1=uint8  SampleTime=-1  InputType=[ 7 ]  OutputType=[ 2 ]  FctDeclaration=extern void floatToBytes(real32_T u1,uint8_T* y1);  FctCall=floatToBytes(%u1, *%y1);  OrderingInOutPopup=None
  C Function Call1 : dsPICdrivers/OTHERS/C Function Call  Tag=dsPIC_dsPIC_CFunctionCall  fctName='floatToBytes'  INPUT_SIZE=1  INPUT1=real32  INPUT2=--  INPUT3=--  OUTPUT_SIZE=4  OUTPUT1=uint8  SampleTime=-1  InputType=[ 7 ]  OutputType=[ 2 ]  FctDeclaration=extern void floatToBytes(real32_T u1,uint8_T* y1);  FctCall=floatToBytes(%u1, *%y1);  OrderingInOutPopup=None
  C Function Call2 : dsPICdrivers/OTHERS/C Function Call  Tag=dsPIC_dsPIC_CFunctionCall  fctName='shortToBytes'  INPUT_SIZE=1  INPUT1=int16  INPUT2=--  INPUT3=--  OUTPUT_SIZE=2  OUTPUT1=uint8  SampleTime=-1  InputType=[ 3 ]  OutputType=[ 2 ]  FctDeclaration=extern void shortToBytes(int16_T u1,uint8_T* y1);  FctCall=shortToBytes(%u1, *%y1);  OrderingInOutPopup=None
  Pack : xpclib/UDP/Pack  datatypes={'uint16', 'uint16', 'uint16', 'uint16', 'uint16', 'uint16', 'uint16', 'uint16', 'uint16',}  byteAlign=1
  Sensor Suite : Subsystem
  myMux Fun : Stateflow chart
  Power : Outport
  Raw Sensors : Outport  Port=2
  Accel : Outport  Port=3
  Gyro : Outport  Port=4
  Dyn : Outport  Port=5
  Mag : Outport  Port=6
  Baro Alt : Outport  Port=7
  Therm Log : Outport  Port=8
  wires:
  Sensor Suite/1(Gyro X) -> Pack/1
  Sensor Suite/2(Gyro Y) -> Pack/2
  Sensor Suite/3(Gyro Z) -> Pack/3
  Sensor Suite/4(Accel X) -> Pack/4
  Sensor Suite/5(Accel Y) -> Pack/5
  Sensor Suite/6(Accel Z) -> Pack/6
  Sensor Suite/7(Mag X) -> Pack/7
  Sensor Suite/8(Mag Y) -> Pack/8
  Sensor Suite/9(Mag Z) -> Pack/9
  Pack/1 -> Raw Sensors/1
  Sensor Suite/13(Accel) -> Accel/1
  Sensor Suite/14(Gyro) -> Gyro/1
  Sensor Suite/15(Power) -> Power/1
  C Function Call/1 -> myMux Fun/1(u1)
  C Function Call1/1 -> myMux Fun/2(u2)
  C Function Call2/1 -> myMux Fun/3(u3)
  Sensor Suite/12(Therm) -> C Function Call2/1
  myMux Fun/1(y) -> Dyn/1
  Sensor Suite/10(Pitot) -> C Function Call/1
  Sensor Suite/11(Static) -> C Function Call1/1
  Sensor Suite/16(Mag) -> Mag/1
  Sensor Suite/17(Baro Alt) -> Baro Alt/1
  Sensor Suite/18(Therm Log) -> Therm Log/1
  D2/1 -> Sensor Suite/1(D2)
  Raw HIL/1 -> Sensor Suite/2(Raw HIL)

== system sensorMCU/To Control  MCU/IPC Data ==
  To SPI : Inport
  Constant1 : Constant  Value=0  OutDataTypeMode=boolean  SampleTime=.01
  Constant2 : Constant  OutDataTypeMode=boolean
  Data Logger1 : dsPICdrivers/OTHERS/C Function Call  Tag=dsPIC_dsPIC_CFunctionCall  fctName='spiSend'  INPUT_SIZE=99  INPUT1=uint8  INPUT2=--  INPUT3=--  OUTPUT_SIZE=1  OUTPUT1=--  SampleTime=-1  InputType=[ 2 ]  OutputType=[ ]  FctDeclaration=extern void spiSend(uint8_T* u1);  FctCall=spiSend(*%u1);  OrderingInOutPopup=Input & Output
  Drive SSL High : dsPICdrivers/Digital I//O/Digital Output Write  Tag=dsPIC_Digital_Output  Orientation=left  Priority=5  PORT=B  Pin=[ 2]  Simultaneous=off  OrderingInOutPopup=Input
  Drive SSL Low : dsPICdrivers/Digital I//O/Digital Output Write  Tag=dsPIC_Digital_Output  Orientation=left  Priority=5  PORT=B  Pin=[ 2]  Simultaneous=off  OrderingInOutPopup=Output
  Nop : dsPICdrivers/OTHERS/Nop  Tag=dsPIC_Reset  Orientation=up  NbrNop=10
  Nop1 : dsPICdrivers/OTHERS/Nop  Tag=dsPIC_Reset  Orientation=up  NbrNop=10
  wires:
  Constant1/1 -> Drive SSL Low/1
  Drive SSL Low/1 -> Nop/1
  Constant2/1 -> Drive SSL High/1
  Data Logger1/1 -> Nop1/1
  To SPI/1 -> Data Logger1/1
  Nop/1 -> Data Logger1/2
  Nop1/1 -> Drive SSL High/2

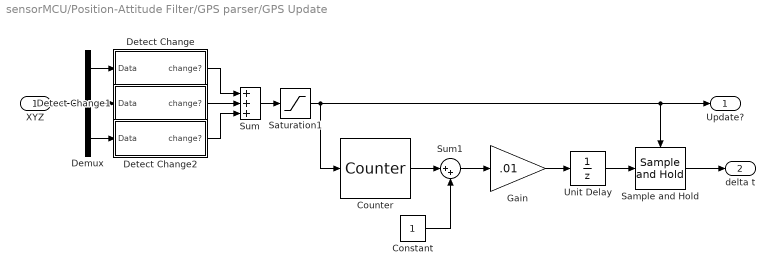
== system sensorMCU/Position-Attitude Filter/GPS parser/GPS Update ==
  XYZ : Inport
  Constant : Constant
  Counter : dspswit3/Counter  Direction=Up  CountEvent=Free running  CounterSize=32 bits  MaxCount=255  InitialCount=0  Output=Count  HitValue=32  ResetInput=on  SamplesPerFrame=1  Ts=-1  CntDtype=double  HitDtype=Logical
  Demux : Demux  Outputs=3
  Detect Change : Subsystem
  Detect Change1 : Subsystem
  Detect Change2 : Subsystem
  Gain : Gain  Gain=.01
  Sample and Hold : dspsigops/Sample and Hold  SystemSampleTime=-1  trig=Rising edge  initCond=10  latchinput=off
  Saturation1 : Saturate  UpperLimit=1  LowerLimit=0
  Sum : Sum  Inputs=3
  Sum1 : Sum  Inputs=|++
  Unit Delay : UnitDelay  X0=10  SampleTime=-1
  Update? : Outport
  delta t : Outport  Port=2
  wires:
  Demux/1 -> Detect Change/1(Data)
  Demux/2 -> Detect Change1/1(Data)
  Demux/3 -> Detect Change2/1(Data)
  Detect Change/1(change?) -> Sum/1
  Detect Change1/1(change?) -> Sum/2
  Detect Change2/1(change?) -> Sum/3
  Sum/1 -> Saturation1/1
  XYZ/1 -> Demux/1
  Saturation1/1 -> Update?/1, Sample and Hold/Trigger, Counter/1
  Sample and Hold/1 -> delta t/1
  Gain/1 -> Unit Delay/1
  Unit Delay/1 -> Sample and Hold/1
  Counter/1 -> Sum1/1
  Sum1/1 -> Gain/1
  Constant/1 -> Sum1/2

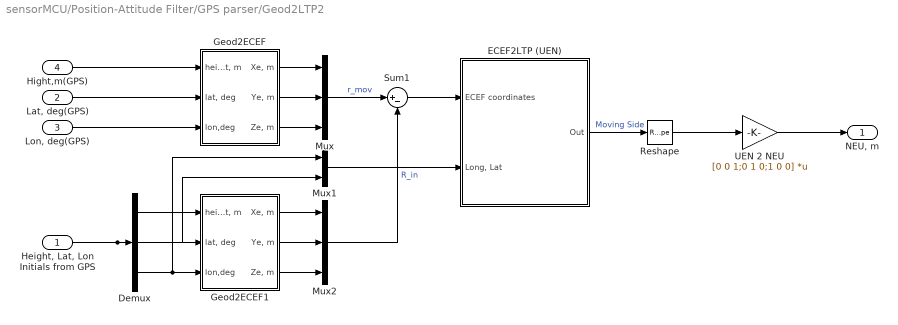
== system sensorMCU/Position-Attitude Filter/GPS parser/Geod2LTP2 ==
  "Height, Lat, Lon Initials from GPS" : Inport
  "Lat, deg(GPS)" : Inport  Port=2
  "Lon, deg(GPS)" : Inport  Port=3
  Hight,m(GPS) : Inport  Port=4
  Demux : Demux  Outputs=3
  ECEF2LTP (UEN) : Subsystem
      mask Display: plot(0,0,100,100,[45,40,35,40,40],[85,95,85,95,40],[85,95,85,95,40],[35,40,45,40,40],[60,40,10,20,10,14],[70,40,10,13,10,20],[56,45],[70,70],[60,60],[50,60],[60,60],[30,40],[50,60],[20,20],[30,40],[20,20],[45,55],[35,25],[75,65],[35,25])
  Geod2ECEF : Subsystem  mask{Re=6378137, Rp=6356752.3142}
      mask prompts: Re "Enter equatorial radius, m"; Rp "Enter polar radius,m"
  Geod2ECEF1 : Subsystem  mask{Re=6378137, Rp=6356752.3142}
      mask prompts: Re "Enter equatorial radius, m"; Rp "Enter polar radius,m"
  Mux : Mux  Inputs=3
  Mux1 : Mux  Inputs=2
  Mux2 : Mux  Inputs=3
  Reshape : Reshape  OutputDimensionality=Column vector (2-D)
  Sum1 : Sum  Inputs=|+-  SaturateOnIntegerOverflow=on
  UEN 2 NEU : Gain  Gain=[0 0 1;0 1 0;1 0 0]  Multiplication=Matrix(K*u)  SaturateOnIntegerOverflow=on
  "NEU, m" : Outport
  wires:
  UEN 2 NEU/1 -> "NEU, m"/1
  Geod2ECEF/3("Ze, m ") -> Mux/3
  Geod2ECEF/1("Xe, m ") -> Mux/1
  Geod2ECEF/2("Ye, m ") -> Mux/2
  "Lat, deg(GPS)"/1 -> Geod2ECEF/2("lat, deg")
  "Lon, deg(GPS)"/1 -> Geod2ECEF/3(lon,deg)
  Mux1/1 -> ECEF2LTP (UEN)/2("Long, Lat")
  Geod2ECEF1/3("Ze, m ") -> Mux2/3
  Geod2ECEF1/1("Xe, m ") -> Mux2/1
  Geod2ECEF1/2("Ye, m ") -> Mux2/2
  Mux2/1 -> Sum1/2  "R_in"
  Demux/1 -> Geod2ECEF1/1("height, m")
  Demux/2 -> Mux1/2, Geod2ECEF1/2("lat, deg")
  Demux/3 -> Mux1/1, Geod2ECEF1/3(lon,deg)
  ECEF2LTP (UEN)/1(Out) -> Reshape/1  "Moving Side"
  Hight,m(GPS)/1 -> Geod2ECEF/1("height, m")
  "Height, Lat, Lon Initials from GPS"/1 -> Demux/1
  Mux/1 -> Sum1/1  "r_mov"
  Sum1/1 -> ECEF2LTP (UEN)/1(ECEF coordinates)
  Reshape/1 -> UEN 2 NEU/1

== system sensorMCU/Position-Attitude Filter/Select HIL or  Live/TimeStamp1 ==
  Ts : Inport
  C Function Call : dsPICdrivers/OTHERS/C Function Call  Tag=dsPIC_dsPIC_CFunctionCall  fctName='uShortToBytes'  INPUT_SIZE=1  INPUT1=uint16  INPUT2=--  INPUT3=--  OUTPUT_SIZE=2  OUTPUT1=uint8  SampleTime=-1  InputType=[ 4 ]  OutputType=[ 2 ]  FctDeclaration=extern void uShortToBytes(uint16_T u1,uint8_T* y1);  FctCall=uShortToBytes(%u1, *%y1);  OrderingInOutPopup=None
  Data Type Conversion5 : DataTypeConversion  OutDataTypeMode=uint16
  Ts bytes : Outport
  wires:
  Data Type Conversion5/1 -> C Function Call/1
  Ts/1 -> Data Type Conversion5/1
  C Function Call/1 -> Ts bytes/1

== system sensorMCU/Position-Attitude Filter/Select HIL or  Live/to Bytes1 ==
  Float : Inport
  C Function Call : dsPICdrivers/OTHERS/C Function Call  Tag=dsPIC_dsPIC_CFunctionCall  fctName='floatToBytes'  INPUT_SIZE=1  INPUT1=real32  INPUT2=--  INPUT3=--  OUTPUT_SIZE=4  OUTPUT1=uint8  SampleTime=-1  InputType=[ 7 ]  OutputType=[ 2 ]  FctDeclaration=extern void floatToBytes(real32_T u1,uint8_T* y1);  FctCall=floatToBytes(%u1, *%y1);  OrderingInOutPopup=None
  C Function Call1 : dsPICdrivers/OTHERS/C Function Call  Tag=dsPIC_dsPIC_CFunctionCall  fctName='floatToBytes'  INPUT_SIZE=1  INPUT1=real32  INPUT2=--  INPUT3=--  OUTPUT_SIZE=4  OUTPUT1=uint8  SampleTime=-1  InputType=[ 7 ]  OutputType=[ 2 ]  FctDeclaration=extern void floatToBytes(real32_T u1,uint8_T* y1);  FctCall=floatToBytes(%u1, *%y1);  OrderingInOutPopup=None
  C Function Call2 : dsPICdrivers/OTHERS/C Function Call  Tag=dsPIC_dsPIC_CFunctionCall  fctName='floatToBytes'  INPUT_SIZE=1  INPUT1=real32  INPUT2=--  INPUT3=--  OUTPUT_SIZE=4  OUTPUT1=uint8  SampleTime=-1  InputType=[ 7 ]  OutputType=[ 2 ]  FctDeclaration=extern void floatToBytes(real32_T u1,uint8_T* y1);  FctCall=floatToBytes(%u1, *%y1);  OrderingInOutPopup=None
  Data Type Conversion : DataTypeConversion  OutDataTypeMode=single
  Demux : Demux  Outputs=3
  Mux : Mux  Inputs=3
  Bytes : Outport
  wires:
  Float/1 -> Data Type Conversion/1
  Demux/1 -> C Function Call/1
  Mux/1 -> Bytes/1
  C Function Call/1 -> Mux/1
  Demux/2 -> C Function Call1/1
  Demux/3 -> C Function Call2/1
  C Function Call1/1 -> Mux/2
  C Function Call2/1 -> Mux/3
  Data Type Conversion/1 -> Demux/1

== system sensorMCU/Position-Attitude Filter/Select HIL or  Live/to Bytes2 ==
  Float : Inport
  C Function Call : dsPICdrivers/OTHERS/C Function Call  Tag=dsPIC_dsPIC_CFunctionCall  fctName='floatToBytes'  INPUT_SIZE=1  INPUT1=real32  INPUT2=--  INPUT3=--  OUTPUT_SIZE=4  OUTPUT1=uint8  SampleTime=-1  InputType=[ 7 ]  OutputType=[ 2 ]  FctDeclaration=extern void floatToBytes(real32_T u1,uint8_T* y1);  FctCall=floatToBytes(%u1, *%y1);  OrderingInOutPopup=None
  C Function Call1 : dsPICdrivers/OTHERS/C Function Call  Tag=dsPIC_dsPIC_CFunctionCall  fctName='floatToBytes'  INPUT_SIZE=1  INPUT1=real32  INPUT2=--  INPUT3=--  OUTPUT_SIZE=4  OUTPUT1=uint8  SampleTime=-1  InputType=[ 7 ]  OutputType=[ 2 ]  FctDeclaration=extern void floatToBytes(real32_T u1,uint8_T* y1);  FctCall=floatToBytes(%u1, *%y1);  OrderingInOutPopup=None
  C Function Call2 : dsPICdrivers/OTHERS/C Function Call  Tag=dsPIC_dsPIC_CFunctionCall  fctName='floatToBytes'  INPUT_SIZE=1  INPUT1=real32  INPUT2=--  INPUT3=--  OUTPUT_SIZE=4  OUTPUT1=uint8  SampleTime=-1  InputType=[ 7 ]  OutputType=[ 2 ]  FctDeclaration=extern void floatToBytes(real32_T u1,uint8_T* y1);  FctCall=floatToBytes(%u1, *%y1);  OrderingInOutPopup=None
  Data Type Conversion : DataTypeConversion  OutDataTypeMode=single
  Demux : Demux  Outputs=3
  Mux : Mux  Inputs=3
  Bytes : Outport
  wires:
  Data Type Conversion/1 -> Demux/1
  C Function Call2/1 -> Mux/3
  C Function Call1/1 -> Mux/2
  Demux/3 -> C Function Call2/1
  Demux/2 -> C Function Call1/1
  C Function Call/1 -> Mux/1
  Mux/1 -> Bytes/1
  Demux/1 -> C Function Call/1
  Float/1 -> Data Type Conversion/1

== system sensorMCU/Position-Attitude Filter/Select HIL or  Live/to Bytes3 ==
  Float : Inport
  C Function Call : dsPICdrivers/OTHERS/C Function Call  Tag=dsPIC_dsPIC_CFunctionCall  fctName='floatToBytes'  INPUT_SIZE=1  INPUT1=real32  INPUT2=--  INPUT3=--  OUTPUT_SIZE=4  OUTPUT1=uint8  SampleTime=-1  InputType=[ 7 ]  OutputType=[ 2 ]  FctDeclaration=extern void floatToBytes(real32_T u1,uint8_T* y1);  FctCall=floatToBytes(%u1, *%y1);  OrderingInOutPopup=None
  C Function Call1 : dsPICdrivers/OTHERS/C Function Call  Tag=dsPIC_dsPIC_CFunctionCall  fctName='floatToBytes'  INPUT_SIZE=1  INPUT1=real32  INPUT2=--  INPUT3=--  OUTPUT_SIZE=4  OUTPUT1=uint8  SampleTime=-1  InputType=[ 7 ]  OutputType=[ 2 ]  FctDeclaration=extern void floatToBytes(real32_T u1,uint8_T* y1);  FctCall=floatToBytes(%u1, *%y1);  OrderingInOutPopup=None
  C Function Call2 : dsPICdrivers/OTHERS/C Function Call  Tag=dsPIC_dsPIC_CFunctionCall  fctName='floatToBytes'  INPUT_SIZE=1  INPUT1=real32  INPUT2=--  INPUT3=--  OUTPUT_SIZE=4  OUTPUT1=uint8  SampleTime=-1  InputType=[ 7 ]  OutputType=[ 2 ]  FctDeclaration=extern void floatToBytes(real32_T u1,uint8_T* y1);  FctCall=floatToBytes(%u1, *%y1);  OrderingInOutPopup=None
  Data Type Conversion : DataTypeConversion  OutDataTypeMode=single
  Demux : Demux  Outputs=3
  Mux : Mux  Inputs=3
  Bytes : Outport
  wires:
  Data Type Conversion/1 -> Demux/1
  C Function Call2/1 -> Mux/3
  C Function Call1/1 -> Mux/2
  Demux/3 -> C Function Call2/1
  Demux/2 -> C Function Call1/1
  C Function Call/1 -> Mux/1
  Mux/1 -> Bytes/1
  Demux/1 -> C Function Call/1
  Float/1 -> Data Type Conversion/1

== system sensorMCU/Position-Attitude Filter/Select HIL or  Live/to Bytes4 ==
  Float : Inport
  C Function Call : dsPICdrivers/OTHERS/C Function Call  Tag=dsPIC_dsPIC_CFunctionCall  fctName='floatToBytes'  INPUT_SIZE=1  INPUT1=real32  INPUT2=--  INPUT3=--  OUTPUT_SIZE=4  OUTPUT1=uint8  SampleTime=-1  InputType=[ 7 ]  OutputType=[ 2 ]  FctDeclaration=extern void floatToBytes(real32_T u1,uint8_T* y1);  FctCall=floatToBytes(%u1, *%y1);  OrderingInOutPopup=None
  C Function Call1 : dsPICdrivers/OTHERS/C Function Call  Tag=dsPIC_dsPIC_CFunctionCall  fctName='floatToBytes'  INPUT_SIZE=1  INPUT1=real32  INPUT2=--  INPUT3=--  OUTPUT_SIZE=4  OUTPUT1=uint8  SampleTime=-1  InputType=[ 7 ]  OutputType=[ 2 ]  FctDeclaration=extern void floatToBytes(real32_T u1,uint8_T* y1);  FctCall=floatToBytes(%u1, *%y1);  OrderingInOutPopup=None
  C Function Call2 : dsPICdrivers/OTHERS/C Function Call  Tag=dsPIC_dsPIC_CFunctionCall  fctName='floatToBytes'  INPUT_SIZE=1  INPUT1=real32  INPUT2=--  INPUT3=--  OUTPUT_SIZE=4  OUTPUT1=uint8  SampleTime=-1  InputType=[ 7 ]  OutputType=[ 2 ]  FctDeclaration=extern void floatToBytes(real32_T u1,uint8_T* y1);  FctCall=floatToBytes(%u1, *%y1);  OrderingInOutPopup=None
  Data Type Conversion : DataTypeConversion  OutDataTypeMode=single
  Demux : Demux  Outputs=3
  Mux : Mux  Inputs=3
  Bytes : Outport
  wires:
  Float/1 -> Data Type Conversion/1
  Demux/1 -> C Function Call/1
  Mux/1 -> Bytes/1
  C Function Call/1 -> Mux/1
  Demux/2 -> C Function Call1/1
  Demux/3 -> C Function Call2/1
  C Function Call1/1 -> Mux/2
  C Function Call2/1 -> Mux/3
  Data Type Conversion/1 -> Demux/1

== system sensorMCU/Position-Attitude Filter/Select HIL or  Live/to Bytes6 ==
  Float : Inport
  C Function Call : dsPICdrivers/OTHERS/C Function Call  Tag=dsPIC_dsPIC_CFunctionCall  fctName='floatToBytes'  INPUT_SIZE=1  INPUT1=real32  INPUT2=--  INPUT3=--  OUTPUT_SIZE=4  OUTPUT1=uint8  SampleTime=-1  InputType=[ 7 ]  OutputType=[ 2 ]  FctDeclaration=extern void floatToBytes(real32_T u1,uint8_T* y1);  FctCall=floatToBytes(%u1, *%y1);  OrderingInOutPopup=None
  C Function Call1 : dsPICdrivers/OTHERS/C Function Call  Tag=dsPIC_dsPIC_CFunctionCall  fctName='floatToBytes'  INPUT_SIZE=1  INPUT1=real32  INPUT2=--  INPUT3=--  OUTPUT_SIZE=4  OUTPUT1=uint8  SampleTime=-1  InputType=[ 7 ]  OutputType=[ 2 ]  FctDeclaration=extern void floatToBytes(real32_T u1,uint8_T* y1);  FctCall=floatToBytes(%u1, *%y1);  OrderingInOutPopup=None
  C Function Call2 : dsPICdrivers/OTHERS/C Function Call  Tag=dsPIC_dsPIC_CFunctionCall  fctName='floatToBytes'  INPUT_SIZE=1  INPUT1=real32  INPUT2=--  INPUT3=--  OUTPUT_SIZE=4  OUTPUT1=uint8  SampleTime=-1  InputType=[ 7 ]  OutputType=[ 2 ]  FctDeclaration=extern void floatToBytes(real32_T u1,uint8_T* y1);  FctCall=floatToBytes(%u1, *%y1);  OrderingInOutPopup=None
  Data Type Conversion : DataTypeConversion  OutDataTypeMode=single
  Demux : Demux  Outputs=3
  Mux : Mux  Inputs=3
  Bytes : Outport
  wires:
  Data Type Conversion/1 -> Demux/1
  C Function Call2/1 -> Mux/3
  C Function Call1/1 -> Mux/2
  Demux/3 -> C Function Call2/1
  Demux/2 -> C Function Call1/1
  C Function Call/1 -> Mux/1
  Mux/1 -> Bytes/1
  Demux/1 -> C Function Call/1
  Float/1 -> Data Type Conversion/1

== system sensorMCU/Sensor Data/Get GPS/Read GPS ==
  Enable : EnablePort
  Demux : Demux  Outputs=[25 1]
  GPS Read : dsPICdrivers/OTHERS/C Function Call  Tag=dsPIC_dsPIC_CFunctionCall  fctName='gpsRead'  INPUT_SIZE=1  INPUT1=--  INPUT2=--  INPUT3=--  OUTPUT_SIZE=26  OUTPUT1=uint8  SampleTime=.01  InputType=[ ]  OutputType=[ 2 ]  FctDeclaration=extern void gpsRead(uint8_T* y1);  FctCall=gpsRead(*%y1);  OrderingInOutPopup=None
  GPS Sentence Parser : dsPICdrivers/OTHERS/C Function Call  Tag=dsPIC_dsPIC_CFunctionCall  fctName='gpsParse'  INPUT_SIZE=127  INPUT1=uint8  INPUT2=--  INPUT3=--  OUTPUT_SIZE=27  OUTPUT1=uint8  SampleTime=-1  InputType=[ 2 ]  OutputType=[ 2 ]  FctDeclaration=extern void gpsParse(uint8_T* u1,uint8_T* y1);  FctCall=gpsParse(*%u1, *%y1);  OrderingInOutPopup=None
  GPS Sentence Split : dsPICdrivers/OTHERS/C Function Call  Tag=dsPIC_dsPIC_CFunctionCall  fctName='gpsSeparate'  INPUT_SIZE=25  INPUT1=uint8  INPUT2=--  INPUT3=--  OUTPUT_SIZE=127  OUTPUT1=uint8  SampleTime=-1  InputType=[ 2 ]  OutputType=[ 2 ]  FctDeclaration=extern void gpsSeparate(uint8_T* u1,uint8_T* y1);  FctCall=gpsSeparate(*%u1, *%y1);  OrderingInOutPopup=None
  Terminator : Terminator
  Out1 : Outport
  wires:
  GPS Sentence Split/1 -> GPS Sentence Parser/1
  GPS Read/1 -> Demux/1
  Demux/1 -> GPS Sentence Split/1
  Demux/2 -> Terminator/1
  GPS Sentence Parser/1 -> Out1/1
